simulink model "DCmotorDrive"  (R2016a)
settings: Solver=FixedStepAuto  StartTime=0.0  StopTime=50  FixedStep=1/512000  MaxStep=1e-5  MinStep=1e-7  RelTol=1e-3
undefined symbols (not defined in the file): rad, s
libraries: powerlib x20, aerolibconvert2 x1, simulink x1, powerlib_meascontrol x1
settings Model: Creator=mrsmash  LastModifiedBy=mrsmash
settings DebuggingCC: MaxConsecutiveZCsMsg=none

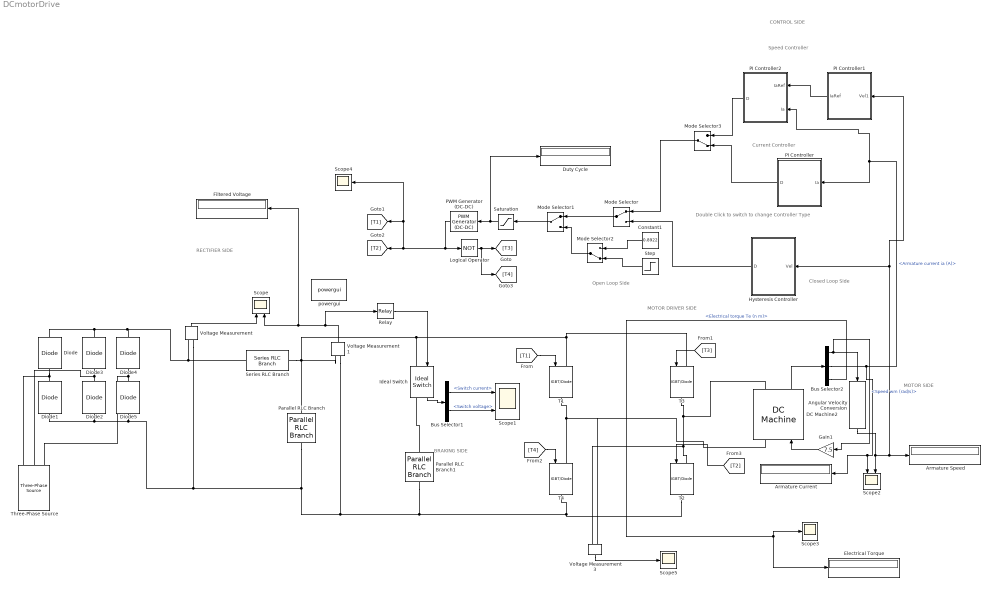
== system DCmotorDrive ==
  note: Open Loop Side
  note: Speed Controller
  note: Current Controller
  note: MOTOR DRIVER SIDE
  note: BRAKING SIDE
  note: CONTROL SIDE
  note: Double Click to switch to change Controller Type
  note: MOTOR SIDE
  note: RECTIFIER SIDE
  note: Closed Loop Side
  Angular Velocity Conversion : aerolibconvert2/Angular Velocity Conversion  IU=rad/s  OU=rpm
  Armature Current : Display
  Armature Speed : Display
  Bus Selector1 : BusSelector  OutputSignals=Switch current,Switch voltage
  Bus Selector2 : BusSelector  OutputSignals=Speed wm (rad/s),Armature current ia (A),Electrical torque Te (n m)
  Constant1 : Constant  Value=0.8922  SampleTime=-1
  DC Machine2 : powerlib/Machines/DC Machine  PresetModel=No  MechanicalLoad=Torque TL  FieldType=Permanent magnet  ShowDetailedParameters=on  MeasurementBus=off  RLa="[0.058  0.004]"  RLf="[ 240  120]"  Laf=1.8  MachineConstant=Torque constant (N.m/A)  Ke=6.68*pi/30  Kt=6.69  J=1240  Bm=0.000001  Tf=0  w0=0  Ifinit=1  TsPowergui=0  TsBlock=-1
  Diode{,1..5} (6 alike) : powerlib/Power Electronics/Diode  Ron=0.001  Lon=0  Vf=0.8  IC=0  UseSnubber=off  Rs=500  Cs=250e-9  Measurements=off
  "Duty Cycle " : Display
  Electrical Torque : Display
  Filtered Voltage : Display
  Gain1 : Gain  Gain=7.5
  Hysteresis Controller : Subsystem
  Ideal Switch : powerlib/Power Electronics/Ideal Switch  Ron=0.000001  Lon=0  IC=0  Rs=1e5  Cs=inf  Measurements=on
  Logical Operator : Logic  Operator=NOT  AllPortsSameDT=off  OutDataTypeStr=boolean
  Mode Selector : ManualSwitch
  Mode Selector1 : ManualSwitch
  Mode Selector2 : ManualSwitch  CurrentSetting=0
  Mode Selector3 : ManualSwitch  CurrentSetting=0
  PI Controller : Subsystem
  PI Controller1 : Subsystem
  PI Controller2 : Subsystem
  PWM Generator (DC-DC) : powerlib_meascontrol/Pulse & Signal Generators/PWM Generator (DC-DC)  Fsw=8000  Ts=0
  Parallel RLC Branch : powerlib/Elements/Parallel RLC Branch  LConnTagsString=a  RConnTagsString=__new0  BranchType=C  Resistance=1  Inductance=1e-3  SetiL0=off  InitialCurrent=0  Capacitance=5e-3  Setx0=on  InitialVoltage=535  Measurements=None
  Parallel RLC Branch1 : powerlib/Elements/Parallel RLC Branch  LConnTagsString=a  RConnTagsString=__new0  BranchType=R  Resistance=0.75  Inductance=1e-3  SetiL0=off  InitialCurrent=0  Capacitance=3.9e-3  Setx0=on  InitialVoltage=535  Measurements=None
  Relay : Relay  OnSwitchValue=725  OffSwitchValue=540
  Saturation : Saturate  UpperLimit=1  LowerLimit=0
  Scope : Scope  NumInputPorts=2
  Scope1 : Scope  NumInputPorts=2
  Scope2 : Scope  NumInputPorts=2
  Scope3 : Scope
  Scope4 : Scope
  Scope5 : Scope
  Series RLC Branch : powerlib/Elements/Series RLC Branch  LConnTagsString=__new0  RConnTagsString=__new0  BranchType=L  Resistance=1  Inductance=1e-3  SetiL0=off  InitialCurrent=0  Capacitance=1e-6  Setx0=off  InitialVoltage=0  Measurements=None
  Step : Step  Time=10  Before=0.8922  After=0.6961  SampleTime=0
  T{1..4} (4 alike) : powerlib/Power Electronics/IGBT//Diode  Ron=1e-3  Rs=1e5  Cs=inf  Measurements=off
  Three-Phase Source : powerlib/Electrical Sources/Three-Phase Source  InternalConnection=Yg  VoltagePhases=on  Voltage=25e3  PhaseAngle=0  Voltage_phases=[398 398 398]/sqrt(3)  PhaseAngles_phases=[0 -120 +120]  Frequency=50  NonIdealSource=off  SpecifyImpedance=off  Resistance=0.8929  Inductance=16.58e-3  ShortCircuitLevel=100e6  BaseVoltage=25e3  XRratio=7  BusType=swing  Pref=10e3  Qref=0  Prefabc=[10e3, 10e3, 10e3]  Qrefabc=[0, 0, 0]  Qmin=-inf  Qmax=inf
  Voltage Measurement : powerlib/Measurements/Voltage Measurement  PhasorSimulation=off  OutputType=Complex  PSBequivalent=0
  Voltage Measurement1 : powerlib/Measurements/Voltage Measurement  PhasorSimulation=off  OutputType=Complex  PSBequivalent=0
  Voltage Measurement3 : powerlib/Measurements/Voltage Measurement  PhasorSimulation=off  OutputType=Complex  PSBequivalent=0
  powergui : powerlib/powergui  Priority=1  SimulationMode=Discrete  SolverType=Tustin/Backward Euler (TBE)  SampleTime=1/512000  frequency=60  SPID=off  DisableSnubberDevices=on  DisableRonSwitches=off  DisableVfSwitches=off  SwTol=0  DisplayEquations=off  Interpol=off  ExternalGateDelay=off  methode=off  Ts=10  FunctionMessages=off  echomessages=off  HookPort=off  EnableUseOfTLC=off  x0status=blocks  frequencyindice=0  Pbase=100e6  ErrMax=1e-4  Iterations=50  UnitsV=kV  UnitsW=MW  buscounter=0  RestoreLinks=warning  ResistiveCurrentMeasurement=off  Frange=[0:2:500]  Ylog=off  Xlog=on  ShowGrid=off  save=off  variable=ZData  structure=0  ZoomFFT=off  StartTime=0.0  cycles=1  DisplayStyle=1  fundamental=60  FreqAxis=off  MaxFrequency=1000  frequencyindicesteady=1  RmsSteady=1  display=off
  wires:
  Voltage Measurement/1 -> Scope/1
  Voltage Measurement1/1 -> Relay/1, Filtered Voltage/1, Scope/2
  DC Machine2/1 -> Bus Selector2/1
  Bus Selector2/1 -> Gain1/1, Angular Velocity Conversion/1  "<Speed wm (rad/s)>"
  Angular Velocity Conversion/1 -> PI Controller1/1(Vel1), Hysteresis Controller/1(Vel), Armature Speed/1, Scope2/2
  Bus Selector2/3 -> Electrical Torque/1, Scope3/1  "<Electrical torque Te (n m)>"
  Bus Selector2/2 -> PI Controller2/2(Ia), PI Controller/1(Ia), Armature Current/1, Scope2/1  "<Armature current ia (A)>"
  [T1] -> T1/1
  [T3] -> T3/1
  [T4] -> T4/1
  [T2] -> T2/1
  Hysteresis Controller/1(D) -> Mode Selector/2
  PWM Generator (DC-DC)/1 -> [T1], Scope4/1, [T2], Logical Operator/1
  Logical Operator/1 -> [T4], [T3]
  Mode Selector/1 -> Mode Selector1/1
  Mode Selector1/1 -> Saturation/1
  Gain1/1 -> DC Machine2/1
  Voltage Measurement3/1 -> Scope5/1
  Mode Selector2/1 -> Mode Selector1/2
  Constant1/1 -> Mode Selector2/1
  Step/1 -> Mode Selector2/2
  Relay/1 -> Ideal Switch/1
  Ideal Switch/1 -> Bus Selector1/1
  Bus Selector1/1 -> Scope1/1  "<Switch current>"
  Bus Selector1/2 -> Scope1/2  "<Switch voltage>"
  Mode Selector3/1 -> Mode Selector/1
  PI Controller/1(D) -> Mode Selector3/2
  PI Controller1/1(IaRef) -> PI Controller2/1(IaRef)
  PI Controller2/1(D) -> Mode Selector3/1
  Saturation/1 -> "Duty Cycle "/1, PWM Generator (DC-DC)/1
  connections:
  T4/LConn1 -- DC Machine2/LConn1 -- Voltage Measurement3/LConn1 -- T1/RConn1
  T3/RConn1 -- Voltage Measurement3/LConn2 -- T2/LConn1 -- DC Machine2/RConn1
  Diode1/RConn1 -- Three-Phase Source/RConn1 -- Diode/LConn1
  Series RLC Branch/LConn1 -- Diode4/RConn1 -- Diode/RConn1 -- Diode3/RConn1 -- Voltage Measurement/LConn1
  Diode3/LConn1 -- Three-Phase Source/RConn2 -- Diode2/RConn1
  Diode4/LConn1 -- Three-Phase Source/RConn3 -- Diode5/RConn1
  Parallel RLC Branch1/LConn1 -- Ideal Switch/RConn1
  Series RLC Branch/RConn1 -- Voltage Measurement1/LConn1 -- Ideal Switch/LConn1 -- T1/LConn1 -- T3/LConn1 -- Parallel RLC Branch/LConn1
  Parallel RLC Branch/RConn1 -- Voltage Measurement1/LConn2 -- Parallel RLC Branch1/RConn1 -- T2/RConn1 -- T4/RConn1 -- Voltage Measurement/LConn2 -- Diode5/LConn1 -- Diode1/LConn1 -- Diode2/LConn1

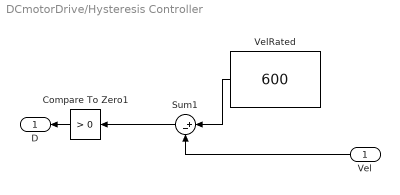
== system DCmotorDrive/Hysteresis Controller ==
  Vel : Inport
  Compare To Zero1 : simulink/Logic and Bit Operations/Compare To Zero  relop=>  OutDataTypeStr=boolean
  Sum1 : Sum  Inputs=|+-
  VelRated : Constant  Value=600  SampleTime=-1
  D : Outport
  wires:
  Compare To Zero1/1 -> D/1
  Vel/1 -> Sum1/2
  VelRated/1 -> Sum1/1
  Sum1/1 -> Compare To Zero1/1

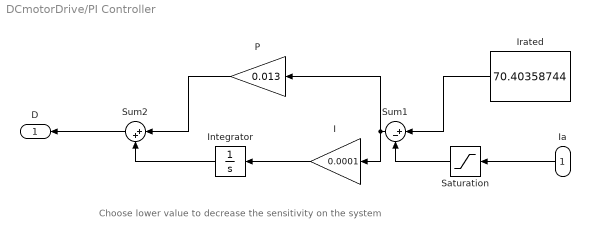
== system DCmotorDrive/PI Controller ==
  note: Choose lower value to decrease the sensitivity on the system
  Ia : Inport
  I : Gain  Gain=0.0001
  Integrator : Integrator
  Irated : Constant  Value=70.40358744  SampleTime=-1
  P : Gain  Gain=0.013
  Saturation : Saturate  UpperLimit=789.6860986547*1.5
  Sum1 : Sum  Inputs=|+-
  Sum2 : Sum  Inputs=|++
  D : Outport
  wires:
  Ia/1 -> Saturation/1
  P/1 -> Sum2/1
  I/1 -> Integrator/1
  Sum1/1 -> P/1, I/1
  Sum2/1 -> D/1
  Integrator/1 -> Sum2/2
  Irated/1 -> Sum1/1
  Saturation/1 -> Sum1/2

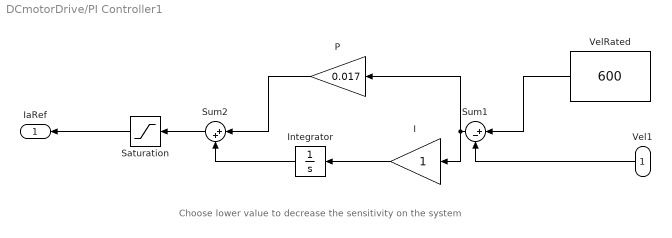
== system DCmotorDrive/PI Controller1 ==
  note: Choose lower value to decrease the sensitivity on the system
  Vel1 : Inport
  I : Gain
  Integrator : Integrator
  P : Gain  Gain=0.017
  Saturation : Saturate  UpperLimit=789.6860986547*1.5
  Sum1 : Sum  Inputs=|+-
  Sum2 : Sum  Inputs=|++
  VelRated : Constant  Value=600  SampleTime=-1
  IaRef : Outport
  wires:
  Vel1/1 -> Sum1/2
  VelRated/1 -> Sum1/1
  Integrator/1 -> Sum2/2
  Sum2/1 -> Saturation/1
  Sum1/1 -> I/1, P/1
  I/1 -> Integrator/1
  P/1 -> Sum2/1
  Saturation/1 -> IaRef/1

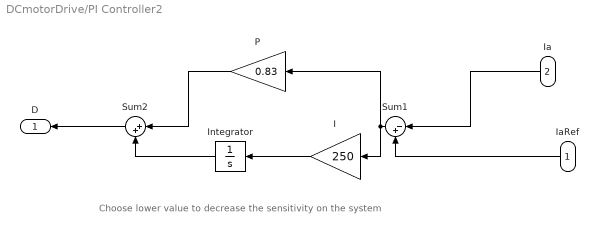
== system DCmotorDrive/PI Controller2 ==
  note: Choose lower value to decrease the sensitivity on the system
  IaRef : Inport
  Ia : Inport  Port=2
  I : Gain  Gain=250
  Integrator : Integrator
  P : Gain  Gain=0.83
  Sum1 : Sum  Inputs=|-+
  Sum2 : Sum  Inputs=|++
  D : Outport
  wires:
  IaRef/1 -> Sum1/2
  Ia/1 -> Sum1/1
  Integrator/1 -> Sum2/2
  Sum2/1 -> D/1
  Sum1/1 -> I/1, P/1
  I/1 -> Integrator/1
  P/1 -> Sum2/1
